simulink model "test02"  (R2026a)
settings: Solver=VariableStepAuto
values from neighbouring files (symbols this model uses):
  K_BB = (R^2 * m * g * d) / (L * (m * R^2 + J))    (= 0.424676496462)    [bnbInit.m]
settings Model: Creator=user  LastModifiedBy=user

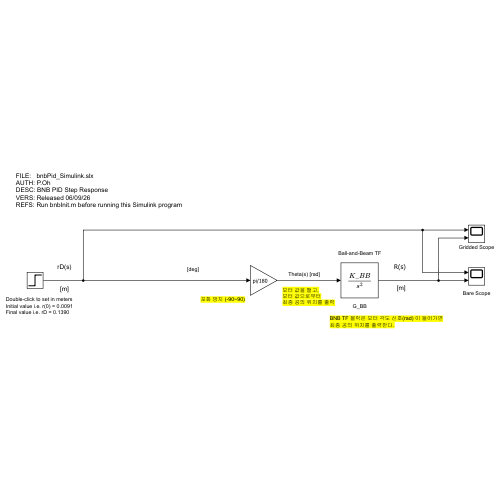
[thumbnail: Simulink's stored preview of the top-level diagram]
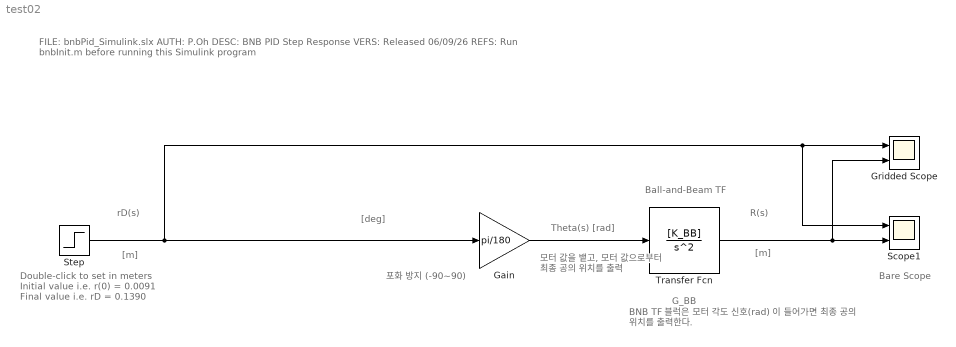
== system test02 ==
  note: Bare Scope
  note: 모터 값을 뱉고,
      | 모터 값으로부터
      | 최종 공의 위치를 출력
  note: 포화 방지 (-90~90)
  note: Double-click to set in meters
      | Initial value i.e. r(0) = 0.0091
      | Final value i.e. rD = 0.1390
  note: R(s)
  note: [m]
  note: G_BB
  note: FILE: bnbPid_Simulink.slx
      | AUTH: P.Oh
      | DESC: BNB PID Step Response
      | VERS: Released 06/09/26
      | REFS: Run bnbInit.m before running this Simulink program
  note: [deg]
  note: Theta(s) [rad]
  note: [m]
  note: Ball-and-Beam TF
  note: rD(s)
  note: BNB TF 블럭은 모터 각도 신호(rad) 이 들어가면
      | 최종 공의 위치를 출력한다.
  Gain : Gain  Gain=pi/180
  Gridded Scope : Scope  NumInputPorts=2
      settings: SampleTime=0.02  ActiveDisplayYMinimum=-0.37499999999999989  ActiveDisplayYMaximum=3.375
  Scope1 : Scope  NumInputPorts=2
      settings: ActiveDisplayYMinimum=-0.027282275035775492  ActiveDisplayYMaximum=0.24554047532197948
  Step : Step  Time=1.0  InitialValue=3  FinalValue=3  SampleTime=0.020
  Transfer Fcn : TransferFcn  Numerator=[K_BB]  Denominator=[1 0 0]
  wires:
  Gain/1 -> Transfer Fcn/1
  Step/1 -> Gain/1, Scope1/1, Gridded Scope/1
  Transfer Fcn/1 -> Gridded Scope/2, Scope1/2
